simulink model "seminar_simulink"  (R2023b)
settings: Solver=VariableStepAuto  StartTime=0.0  StopTime=18000  RelTol=1e-3
settings Model: Creator=64190102  LastModifiedBy=matej
settings SolverCC: AlgebraicLoopSolver=TrustRegion
settings DebuggingCC: UnconnectedInputMsg=warning  UnconnectedOutputMsg=warning  UnconnectedLineMsg=warning
settings ModelReferenceCC: EnableRefExpFcnMdlSchedulingChecks=on
settings RTWCC: DLArmComputeVersion=19.05

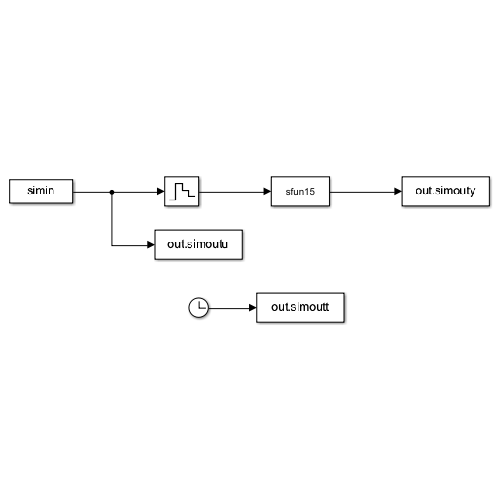
[thumbnail: Simulink's stored preview of the top-level diagram]
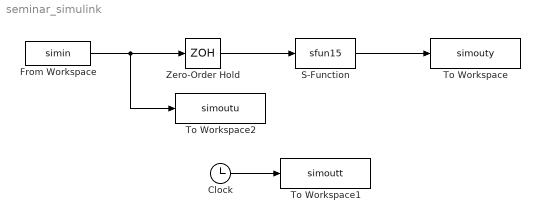
== system seminar_simulink ==
  Clock : Clock
  From Workspace : FromWorkspace  VariableName=simin  SampleTime=16
  S-Function : S-Function  FunctionName=sfun15  SFunctionDeploymentMode=off  EnableBusSupport=off
  To Workspace : ToWorkspace  VariableName=simouty  SaveFormat=Timeseries  SampleTime=16
  To Workspace1 : ToWorkspace  VariableName=simoutt  SaveFormat=Timeseries  SampleTime=16
  To Workspace2 : ToWorkspace  VariableName=simoutu  SaveFormat=Timeseries  SampleTime=16
  Zero-Order Hold : ZeroOrderHold  SampleTime=16
  wires:
  Zero-Order Hold/1 -> S-Function/1
  S-Function/1 -> To Workspace/1
  Clock/1 -> To Workspace1/1
  From Workspace/1 -> To Workspace2/1, Zero-Order Hold/1
